simulink model "receiver"  (R2020b)
settings: Solver=VariableStepAuto  StartTime=0.0  StopTime=10000/3.2e6  RelTol=1e-3
PreLoadFcn:
  | setup_receiver
InitFcn:
  | setup_receiver
undefined symbols (not defined in the file): AXI4, designMultirateFIR, fir_bbuf, Lite, tx_data, xlfda_numerator
libraries: xbsIndex_r4 x428, hdlsllib x13, dspmlti4 x8, xrbsSSR_Library x6, dspswit3 x4, commrandsrc3 x2, dspsigops x2, simulink x1
(part 3 of 5)

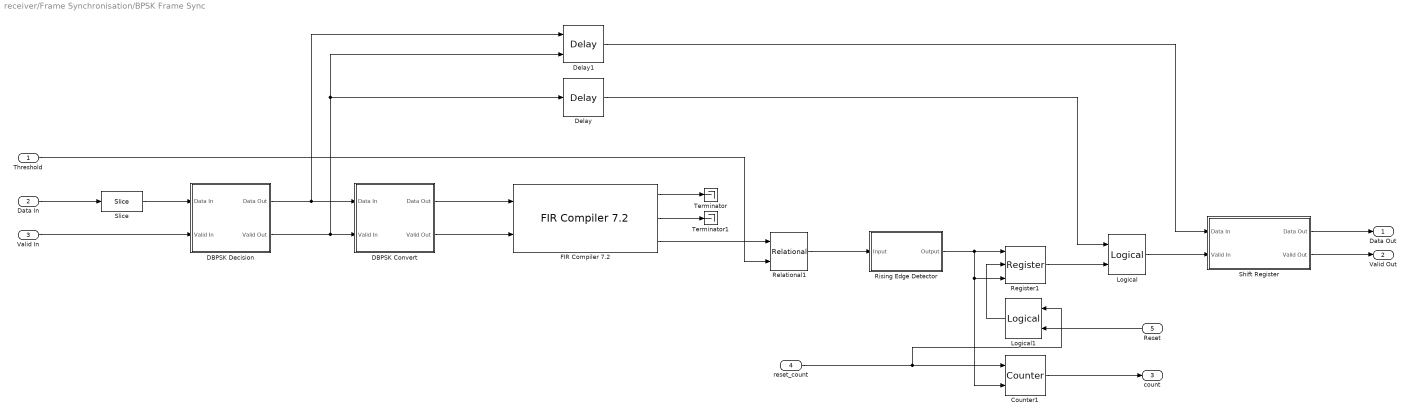
== system receiver/Frame Synchronisation/BPSK Frame Sync ==
  Threshold : Inport
  Data In : Inport  Port=2
  Valid In : Inport  Port=3
  reset_count : Inport  Port=4
  Reset : Inport  Port=5
  Counter1 : xbsIndex_r4/Counter  cnt_type=Free Running  cnt_to=Inf  operation=Up  start_count=0  cnt_by_val=1  arith_type=Unsigned  n_bits=32  bin_pt=0  load_pin=off  rst=on  en=on  explicit_period=off  period=1  use_behavioral_HDL=off  implementation=Fabric  dbl_ovrd=off  block_type=counter
  DBPSK Convert : Subsystem
  DBPSK Decision : Subsystem
  Delay : xbsIndex_r4/Delay  rst=off  infoeditControl=Selection of Reset will increase slice count due to use of real FFs and instead of SRLs  en=off  latency=2  reg_retiming=off  dbl_ovrd=off  block_type=delay
  Delay1 : xbsIndex_r4/Delay  rst=off  infoeditControl=Selection of Reset will increase slice count due to use of real FFs and instead of SRLs  en=on  latency=2  reg_retiming=off  dbl_ovrd=off  block_type=delay
  "FIR Compiler 7.2 " : xbsIndex_r4/FIR Compiler 7.2   coefficientvector=fliplr(double(fir_bbuf))  coefficient_sets=1  coefficient_reload=off  filter_type=Single_Rate  rate_change_type=Integer  interpolation_rate=1  decimation_rate=1  zero_pack_factor=1  channel_sequence=Basic  number_channels=1  pattern_list='P4-0,P4-1,P4-2,P4-3,P4-4'  number_paths=1  ratespecification=Maximum_Possible  sampleperiod=40  hardwareoversamplingrate=1  coefficient_sign=Signed  quantization=Integer_Coefficients  coefficient_width=2  bestprecision=off  coefficient_fractional_bits=0  coefficient_structure=Inferred  output_rounding_mode=Full_Precision  output_width=22  filter_architecture=Systolic_Multiply_Accumulate  optimization_goal=Area  optimization_list='None'  data_buffer_type=Automatic  coefficient_buffer_type=Automatic  input_buffer_type=Automatic  output_buffer_type=Automatic  preference_for_other_storage=Automatic  multi_column_support=Automatic  columnconfig='39'  inter_column_pipe_length=4  data_has_tlast=Not_Required  m_data_has_tready=off  s_data_has_fifo=off  s_data_has_tuser=Not_Required  m_data_has_tuser=Not_Required  s_config_sync_mode=On_Vector  s_config_method=Single  num_reload_slots=1  has_aclken=on  has_aresetn=off  infoeditControl=ARESETn must be asserted for a minimum of 2 cycles  reset_data_vector=on  trim_axipin_name=on  simulation_type=hybrid_sim  simulation_model=sysgen:xfirv7_2_cmodel  data_path_portlist={ 's_axis_data_tdata', 'm_axis_data_tdata' }  passband_min=0.0  passband_max=0.5  stopband_min=0.5  stopband_max=1.0  filter_selection=1  gui_behaviour='Sysgen_GUI'  data_sign=Signed  data_width=16  data_fractional_bits=0  data_tuser_width=1  wrapper_available=true  ip_wrap_arbitrary_binary_point=true  ip_name=FIR Compiler  ip_version=7.2  dsptool_ready=true  ipcore_usecache=true  ipcore_useipmodelcache=true  port_translation_map={ 'aclken' => 'en', 'aresetn' => 'rst' }  run_core_at_system_period=true  ipcore_xco_need_fpga_part=true  block_type=fir_compiler_v7_2
      settings: infoedit=Maximum Possible : Maximizes oversampling rate. Abstracted input handshake (no s_data_tvalid) and automatic rate propagation.<br>Hardware Oversampling Rate : Specifies oversampling rate relative to the input sample period. Abstracted input handshake (no s_data_tvalid) and automatic rate propagation.<br>Input/Output Sample Period : Specifies absolute oversampling rate. No input handshake abstraction (exposes s_data_tvalid) and no rate propagation.
  Logical : xbsIndex_r4/Logical  logical_function=AND  inputs=2  en=off  latency=0  precision=Full  arith_type=Unsigned  n_bits=16  bin_pt=0  align_bp=on  dbl_ovrd=off  block_type=logical
  Logical1 : xbsIndex_r4/Logical  logical_function=OR  inputs=2  en=off  latency=0  precision=Full  arith_type=Unsigned  n_bits=16  bin_pt=0  align_bp=on  dbl_ovrd=off  block_type=logical
  Register1 : xbsIndex_r4/Register  init=0  rst=on  en=on  dbl_ovrd=off  block_type=register
  Relational1 : xbsIndex_r4/Relational  mode=a>=b  op_type=Bool  en=off  latency=0  dbl_ovrd=off  block_type=relational
  Rising Edge Detector : Subsystem
  Shift Register : Subsystem
  Slice : xbsIndex_r4/Slice  nbits=1  boolean_output=off  mode=Upper Bit Location + Width  bit1=0  base1=MSB of Input  bit0=0  base0=LSB of Input  dbl_ovrd=off  block_type=slice
  Terminator : Terminator
  Terminator1 : Terminator
  Data Out : Outport  VectorParamsAs1DForOutWhenUnconnected=off
  Valid Out : Outport  Port=2  VectorParamsAs1DForOutWhenUnconnected=off
  count : Outport  Port=3  VectorParamsAs1DForOutWhenUnconnected=off
  wires:
  DBPSK Convert/1(Data Out) -> "FIR Compiler 7.2 "/1
  DBPSK Decision/2(Valid Out) -> Delay1/2, Delay/1, DBPSK Convert/2(Valid In)
  Reset/1 -> Logical1/2
  Relational1/1 -> Rising Edge Detector/1(Input)
  DBPSK Decision/1(Data Out) -> Delay1/1, DBPSK Convert/1(Data In)
  Delay1/1 -> Shift Register/1(Data In)
  Logical/1 -> Shift Register/2(Valid In)
  Threshold/1 -> Relational1/2
  Logical1/1 -> Register1/2
  Counter1/1 -> count/1
  Valid In/1 -> DBPSK Decision/2(Valid In)
  Slice/1 -> DBPSK Decision/1(Data In)
  "FIR Compiler 7.2 "/2 -> Terminator1/1
  Rising Edge Detector/1(Output) -> Counter1/2, Register1/3, Register1/1
  Register1/1 -> Logical/2
  Shift Register/1(Data Out) -> Data Out/1
  DBPSK Convert/2(Valid Out) -> "FIR Compiler 7.2 "/2
  "FIR Compiler 7.2 "/1 -> Terminator/1
  reset_count/1 -> Logical1/1, Counter1/1
  "FIR Compiler 7.2 "/3 -> Relational1/1
  Delay/1 -> Logical/1
  Data In/1 -> Slice/1
  Shift Register/2(Valid Out) -> Valid Out/1

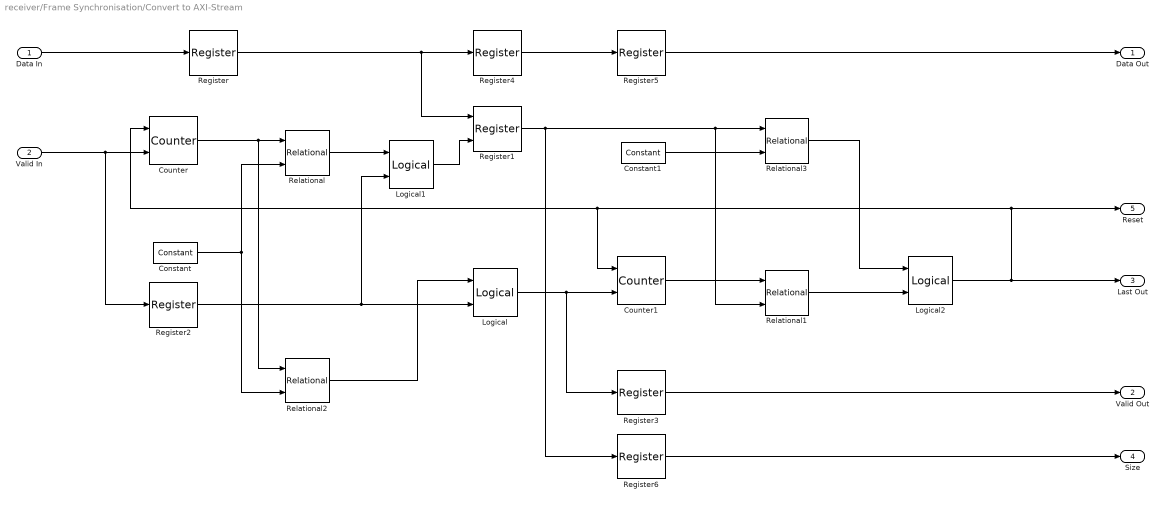
== system receiver/Frame Synchronisation/Convert to AXI-Stream ==
  Data In : Inport
  Valid In : Inport  Port=2
  Constant : xbsIndex_r4/Constant  const=1.0  gui_display_data_type=Fixed-point  arith_type=Unsigned  n_bits=1  bin_pt=0  preci_type=Single  exp_width=8  frac_width=24  explicit_period=off  period=1  equ=P=C  opselect=C  inp2=PCIN>>17  opr=+  inp1=P  carry=CIN  dbl_ovrd=off  block_type=constant
  Constant1 : xbsIndex_r4/Constant  const=0  gui_display_data_type=Fixed-point  arith_type=Unsigned  n_bits=1  bin_pt=0  preci_type=Single  exp_width=8  frac_width=24  explicit_period=off  period=1  equ=P=C  opselect=C  inp2=PCIN>>17  opr=+  inp1=P  carry=CIN  dbl_ovrd=off  block_type=constant
  Counter : xbsIndex_r4/Counter  cnt_type=Free Running  cnt_to=Inf  operation=Up  start_count=0  cnt_by_val=1  arith_type=Unsigned  n_bits=32  bin_pt=0  load_pin=off  rst=on  en=on  explicit_period=off  period=1  use_behavioral_HDL=off  implementation=Fabric  dbl_ovrd=off  block_type=counter
  Counter1 : xbsIndex_r4/Counter  cnt_type=Free Running  cnt_to=Inf  operation=Up  start_count=0  cnt_by_val=1  arith_type=Unsigned  n_bits=32  bin_pt=0  load_pin=off  rst=on  en=on  explicit_period=off  period=1  use_behavioral_HDL=off  implementation=Fabric  dbl_ovrd=off  block_type=counter
  Logical : xbsIndex_r4/Logical  logical_function=AND  inputs=2  en=off  latency=1  precision=Full  arith_type=Unsigned  n_bits=16  bin_pt=0  align_bp=on  dbl_ovrd=off  block_type=logical
  Logical1 : xbsIndex_r4/Logical  logical_function=AND  inputs=2  en=off  latency=0  precision=Full  arith_type=Unsigned  n_bits=16  bin_pt=0  align_bp=on  dbl_ovrd=off  block_type=logical
  Logical2 : xbsIndex_r4/Logical  logical_function=AND  inputs=2  en=off  latency=0  precision=Full  arith_type=Unsigned  n_bits=16  bin_pt=0  align_bp=on  dbl_ovrd=off  block_type=logical
  Register{,2..6} (6 alike) : xbsIndex_r4/Register  init=0  rst=off  en=off  dbl_ovrd=off  block_type=register
  Register1 : xbsIndex_r4/Register  init=0  rst=off  en=on  dbl_ovrd=off  block_type=register
  Relational : xbsIndex_r4/Relational  mode=a=b  op_type=Bool  en=off  latency=0  dbl_ovrd=off  block_type=relational
  Relational1 : xbsIndex_r4/Relational  mode=a>=b  op_type=Bool  en=off  latency=0  dbl_ovrd=off  block_type=relational
  Relational2 : xbsIndex_r4/Relational  mode=a>b  op_type=Bool  en=off  latency=0  dbl_ovrd=off  block_type=relational
  Relational3 : xbsIndex_r4/Relational  mode=a!=b  op_type=Bool  en=off  latency=0  dbl_ovrd=off  block_type=relational
  Data Out : Outport  VectorParamsAs1DForOutWhenUnconnected=off
  Valid Out : Outport  Port=2  VectorParamsAs1DForOutWhenUnconnected=off
  Last Out : Outport  Port=3  VectorParamsAs1DForOutWhenUnconnected=off
  Size : Outport  Port=4  VectorParamsAs1DForOutWhenUnconnected=off
  Reset : Outport  Port=5  VectorParamsAs1DForOutWhenUnconnected=off
  wires:
  Valid In/1 -> Register2/1, Counter/2
  Counter/1 -> Relational2/1, Relational/1
  Data In/1 -> Register/1
  Register/1 -> Register4/1, Register1/1
  Logical/1 -> Register3/1, Counter1/2
  Counter1/1 -> Relational1/1
  Register1/1 -> Register6/1, Relational3/1, Relational1/2
  Register2/1 -> Logical1/2, Logical/2
  Register3/1 -> Valid Out/1
  Register4/1 -> Register5/1
  Register5/1 -> Data Out/1
  Constant/1 -> Relational/2, Relational2/2
  Relational2/1 -> Logical/1
  Relational/1 -> Logical1/1
  Logical1/1 -> Register1/2
  Constant1/1 -> Relational3/2
  Relational3/1 -> Logical2/1
  Relational1/1 -> Logical2/2
  Logical2/1 -> Counter/1, Counter1/1, Reset/1, Last Out/1
  Register6/1 -> Size/1

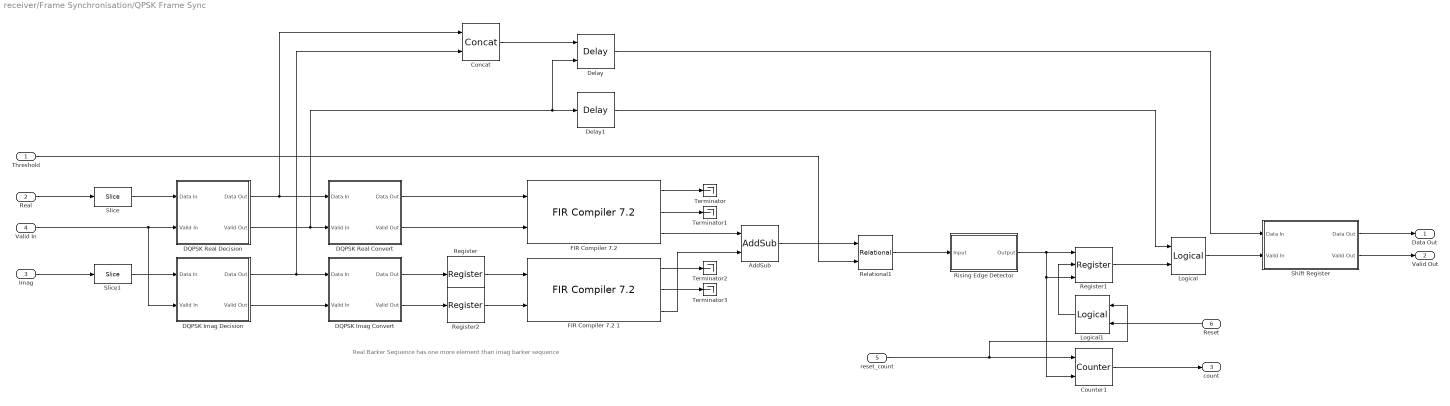
== system receiver/Frame Synchronisation/QPSK Frame Sync ==
  note: Real Barker Sequence has one more element than imag barker sequence
  Threshold : Inport
  Real : Inport  Port=2
  Imag : Inport  Port=3
  Valid In : Inport  Port=4
  reset_count : Inport  Port=5
  Reset : Inport  Port=6
  AddSub : xbsIndex_r4/AddSub  mode=Addition  use_carryin=off  use_carryout=off  en=off  latency=0  precision=Full  arith_type=Unsigned  n_bits=16  bin_pt=14  quantization=Truncate  overflow=Wrap  use_behavioral_HDL=off  hw_selection=Fabric  pipelined=off  dbl_ovrd=off  block_type=addsub
  Concat : xbsIndex_r4/Concat  num_inputs=2  dbl_ovrd=off  block_type=concat
  Counter1 : xbsIndex_r4/Counter  cnt_type=Free Running  cnt_to=Inf  operation=Up  start_count=0  cnt_by_val=1  arith_type=Unsigned  n_bits=32  bin_pt=0  load_pin=off  rst=on  en=on  explicit_period=off  period=1  use_behavioral_HDL=off  implementation=Fabric  dbl_ovrd=off  block_type=counter
  DQPSK Imag Convert : Subsystem
  DQPSK Imag Decision : Subsystem
  DQPSK Real Convert : Subsystem
  DQPSK Real Decision : Subsystem
  Delay : xbsIndex_r4/Delay  rst=off  infoeditControl=Selection of Reset will increase slice count due to use of real FFs and instead of SRLs  en=on  latency=3  reg_retiming=off  dbl_ovrd=off  block_type=delay
  Delay1 : xbsIndex_r4/Delay  rst=off  infoeditControl=Selection of Reset will increase slice count due to use of real FFs and instead of SRLs  en=off  latency=1  reg_retiming=off  dbl_ovrd=off  block_type=delay
  "FIR Compiler 7.2 " : xbsIndex_r4/FIR Compiler 7.2   coefficientvector=fliplr(double(fir_bbuf(1:2:end)))  coefficient_sets=1  coefficient_reload=off  filter_type=Single_Rate  rate_change_type=Integer  interpolation_rate=1  decimation_rate=1  zero_pack_factor=1  channel_sequence=Basic  number_channels=1  pattern_list='P4-0,P4-1,P4-2,P4-3,P4-4'  number_paths=1  ratespecification=Maximum_Possible  sampleperiod=20  hardwareoversamplingrate=1  coefficient_sign=Signed  quantization=Integer_Coefficients  coefficient_width=2  bestprecision=off  coefficient_fractional_bits=0  coefficient_structure=Inferred  output_rounding_mode=Full_Precision  output_width=21  filter_architecture=Systolic_Multiply_Accumulate  optimization_goal=Area  optimization_list='None'  data_buffer_type=Automatic  coefficient_buffer_type=Automatic  input_buffer_type=Automatic  output_buffer_type=Automatic  preference_for_other_storage=Automatic  multi_column_support=Automatic  columnconfig='20'  inter_column_pipe_length=4  data_has_tlast=Not_Required  m_data_has_tready=off  s_data_has_fifo=off  s_data_has_tuser=Not_Required  m_data_has_tuser=Not_Required  s_config_sync_mode=On_Vector  s_config_method=Single  num_reload_slots=1  has_aclken=on  has_aresetn=off  infoeditControl=ARESETn must be asserted for a minimum of 2 cycles  reset_data_vector=on  trim_axipin_name=on  simulation_type=hybrid_sim  simulation_model=sysgen:xfirv7_2_cmodel  data_path_portlist={ 's_axis_data_tdata', 'm_axis_data_tdata' }  passband_min=0.0  passband_max=0.5  stopband_min=0.5  stopband_max=1.0  filter_selection=1  gui_behaviour='Sysgen_GUI'  data_sign=Signed  data_width=16  data_fractional_bits=0  data_tuser_width=1  wrapper_available=true  ip_wrap_arbitrary_binary_point=true  ip_name=FIR Compiler  ip_version=7.2  dsptool_ready=true  ipcore_usecache=true  ipcore_useipmodelcache=true  port_translation_map={ 'aclken' => 'en', 'aresetn' => 'rst' }  run_core_at_system_period=true  ipcore_xco_need_fpga_part=true  block_type=fir_compiler_v7_2
      settings: infoedit=Maximum Possible : Maximizes oversampling rate. Abstracted input handshake (no s_data_tvalid) and automatic rate propagation.<br>Hardware Oversampling Rate : Specifies oversampling rate relative to the input sample period. Abstracted input handshake (no s_data_tvalid) and automatic rate propagation.<br>Input/Output Sample Period : Specifies absolute oversampling rate. No input handshake abstraction (exposes s_data_tvalid) and no rate propagation.
  FIR Compiler 7.2 1 : xbsIndex_r4/FIR Compiler 7.2   coefficientvector=fliplr(double(fir_bbuf(2:2:end)))  coefficient_sets=1  coefficient_reload=off  filter_type=Single_Rate  rate_change_type=Integer  interpolation_rate=1  decimation_rate=1  zero_pack_factor=1  channel_sequence=Basic  number_channels=1  pattern_list='P4-0,P4-1,P4-2,P4-3,P4-4'  number_paths=1  ratespecification=Maximum_Possible  sampleperiod=20  hardwareoversamplingrate=1  coefficient_sign=Signed  quantization=Integer_Coefficients  coefficient_width=2  bestprecision=off  coefficient_fractional_bits=0  coefficient_structure=Inferred  output_rounding_mode=Full_Precision  output_width=21  filter_architecture=Systolic_Multiply_Accumulate  optimization_goal=Area  optimization_list='None'  data_buffer_type=Automatic  coefficient_buffer_type=Automatic  input_buffer_type=Automatic  output_buffer_type=Automatic  preference_for_other_storage=Automatic  multi_column_support=Automatic  columnconfig='19'  inter_column_pipe_length=4  data_has_tlast=Not_Required  m_data_has_tready=off  s_data_has_fifo=off  s_data_has_tuser=Not_Required  m_data_has_tuser=Not_Required  s_config_sync_mode=On_Vector  s_config_method=Single  num_reload_slots=1  has_aclken=on  has_aresetn=off  infoeditControl=ARESETn must be asserted for a minimum of 2 cycles  reset_data_vector=on  trim_axipin_name=on  simulation_type=hybrid_sim  simulation_model=sysgen:xfirv7_2_cmodel  data_path_portlist={ 's_axis_data_tdata', 'm_axis_data_tdata' }  passband_min=0.0  passband_max=0.5  stopband_min=0.5  stopband_max=1.0  filter_selection=1  gui_behaviour='Sysgen_GUI'  data_sign=Signed  data_width=16  data_fractional_bits=0  data_tuser_width=1  wrapper_available=true  ip_wrap_arbitrary_binary_point=true  ip_name=FIR Compiler  ip_version=7.2  dsptool_ready=true  ipcore_usecache=true  ipcore_useipmodelcache=true  port_translation_map={ 'aclken' => 'en', 'aresetn' => 'rst' }  run_core_at_system_period=true  ipcore_xco_need_fpga_part=true  block_type=fir_compiler_v7_2
      settings: infoedit=Maximum Possible : Maximizes oversampling rate. Abstracted input handshake (no s_data_tvalid) and automatic rate propagation.<br>Hardware Oversampling Rate : Specifies oversampling rate relative to the input sample period. Abstracted input handshake (no s_data_tvalid) and automatic rate propagation.<br>Input/Output Sample Period : Specifies absolute oversampling rate. No input handshake abstraction (exposes s_data_tvalid) and no rate propagation.
  Logical : xbsIndex_r4/Logical  logical_function=AND  inputs=2  en=off  latency=0  precision=Full  arith_type=Unsigned  n_bits=16  bin_pt=0  align_bp=on  dbl_ovrd=off  block_type=logical
  Logical1 : xbsIndex_r4/Logical  logical_function=OR  inputs=2  en=off  latency=0  precision=Full  arith_type=Unsigned  n_bits=16  bin_pt=0  align_bp=on  dbl_ovrd=off  block_type=logical
  Register : xbsIndex_r4/Register  init=0  rst=off  en=off  dbl_ovrd=off  block_type=register
  Register1 : xbsIndex_r4/Register  init=0  rst=on  en=on  dbl_ovrd=off  block_type=register
  Register2 : xbsIndex_r4/Register  init=0  rst=off  en=off  dbl_ovrd=off  block_type=register
  Relational1 : xbsIndex_r4/Relational  mode=a>=b  op_type=Bool  en=off  latency=0  dbl_ovrd=off  block_type=relational
  Rising Edge Detector : Subsystem
  Shift Register : Subsystem
  Slice : xbsIndex_r4/Slice  nbits=1  boolean_output=off  mode=Upper Bit Location + Width  bit1=0  base1=MSB of Input  bit0=0  base0=LSB of Input  dbl_ovrd=off  block_type=slice
  Slice1 : xbsIndex_r4/Slice  nbits=1  boolean_output=off  mode=Upper Bit Location + Width  bit1=0  base1=MSB of Input  bit0=0  base0=LSB of Input  dbl_ovrd=off  block_type=slice
  Terminator{,1..3} (4 alike) : Terminator
  Data Out : Outport  VectorParamsAs1DForOutWhenUnconnected=off
  Valid Out : Outport  Port=2  VectorParamsAs1DForOutWhenUnconnected=off
  count : Outport  Port=3  VectorParamsAs1DForOutWhenUnconnected=off
  wires:
  Delay1/1 -> Logical/1
  Delay/1 -> Shift Register/1(Data In)
  Concat/1 -> Delay/1
  Register2/1 -> FIR Compiler 7.2 1/2
  Register/1 -> FIR Compiler 7.2 1/1
  DQPSK Imag Convert/2(Valid Out) -> Register2/1
  DQPSK Imag Convert/1(Data Out) -> Register/1
  FIR Compiler 7.2 1/1 -> Terminator2/1
  FIR Compiler 7.2 1/2 -> Terminator3/1
  FIR Compiler 7.2 1/3 -> AddSub/2
  AddSub/1 -> Relational1/1
  "FIR Compiler 7.2 "/3 -> AddSub/1
  DQPSK Imag Decision/2(Valid Out) -> DQPSK Imag Convert/2(Valid In)
  DQPSK Imag Decision/1(Data Out) -> DQPSK Imag Convert/1(Data In), Concat/2
  Slice1/1 -> DQPSK Imag Decision/1(Data In)
  Imag/1 -> Slice1/1
  DQPSK Real Convert/1(Data Out) -> "FIR Compiler 7.2 "/1
  Reset/1 -> Logical1/2
  Relational1/1 -> Rising Edge Detector/1(Input)
  DQPSK Real Decision/1(Data Out) -> DQPSK Real Convert/1(Data In), Concat/1
  Logical/1 -> Shift Register/2(Valid In)
  Threshold/1 -> Relational1/2
  Logical1/1 -> Register1/2
  Counter1/1 -> count/1
  Valid In/1 -> DQPSK Real Decision/2(Valid In), DQPSK Imag Decision/2(Valid In)
  Slice/1 -> DQPSK Real Decision/1(Data In)
  "FIR Compiler 7.2 "/2 -> Terminator1/1
  Rising Edge Detector/1(Output) -> Counter1/2, Register1/3, Register1/1
  Register1/1 -> Logical/2
  Shift Register/1(Data Out) -> Data Out/1
  DQPSK Real Convert/2(Valid Out) -> "FIR Compiler 7.2 "/2
  "FIR Compiler 7.2 "/1 -> Terminator/1
  reset_count/1 -> Logical1/1, Counter1/1
  DQPSK Real Decision/2(Valid Out) -> DQPSK Real Convert/2(Valid In), Delay1/1, Delay/2
  Real/1 -> Slice/1
  Shift Register/2(Valid Out) -> Valid Out/1

== system receiver/Observation Point/op ==
  Data In : Inport
  Valid In : Inport  Port=2
  Cast To Boolean : DataTypeConversion  OutDataTypeStr=boolean
  Constellation Diagram : ConstellationDiagram
  Convert Protect : DataTypeConversion  OutDataTypeStr=fixdt(0,32,0)  ConvertRealWorld=Stored Integer (SI)
  Delay : Delay  DelayLength=1  ShowEnablePort=on
      settings: InputPortMap=u0,e6
  Imag Conversion : DataTypeConversion  OutDataTypeStr=fixdt(1,16,15)  ConvertRealWorld=Stored Integer (SI)
  Imag Slice : hdlsllib/Logic and Bit Operations/Bit Slice  lidx=31  ridx=16
      settings: SourceProductBaseCode=SL
  Real Conversion : DataTypeConversion  OutDataTypeStr=fixdt(1,16,15)  ConvertRealWorld=Stored Integer (SI)
  Real Slice : hdlsllib/Logic and Bit Operations/Bit Slice  lidx=15  ridx=0
      settings: SourceProductBaseCode=SL
  Real-Imag to Complex : RealImagToComplex
  Time Scope : Scope
  m_axis_op_tdata : xbsIndex_r4/Gateway Out  inherit_from_input=on  hdl_port=on  rows=1  columns=1  UseAsDAC=off  DACChannel='1'  interface=None  automatic_assignment=on  address_offset=hex2dec('00')  intf_name=''  intf_description=''  timing_constraint=None  locs_specified=off  LOCs={}  io_standard={}  block_type=gatewayout
  m_axis_op_tvalid : xbsIndex_r4/Gateway Out  inherit_from_input=on  hdl_port=on  rows=1  columns=1  UseAsDAC=off  DACChannel='1'  interface=None  automatic_assignment=on  address_offset=hex2dec('00')  intf_name=''  intf_description=''  timing_constraint=None  locs_specified=off  LOCs={}  io_standard={}  block_type=gatewayout
  wires:
  Cast To Boolean/1 -> Delay/2
  Convert Protect/1 -> Imag Slice/1, Real Slice/1
  Real-Imag to Complex/1 -> Delay/1
  m_axis_op_tdata/1 -> Convert Protect/1
  Imag Conversion/1 -> Real-Imag to Complex/2
  Imag Slice/1 -> Imag Conversion/1
  Real Slice/1 -> Real Conversion/1
  Real Conversion/1 -> Real-Imag to Complex/1
  m_axis_op_tvalid/1 -> Cast To Boolean/1
  Delay/1 -> Constellation Diagram/1, Time Scope/1
  Data In/1 -> m_axis_op_tdata/1
  Valid In/1 -> m_axis_op_tvalid/1

== system receiver/QPSK System/QPSK TX Generation ==
  Enable : Inport
  Bernoulli Binary Generator : commrandsrc3/Bernoulli Binary Generator  ProbabilityOfZero=0.5  SeedSource=Parameter  Seed=53  SampleTime=1/100e3  SamplesPerFrame=1  OutputDataType=double  SimulateUsing=Interpreted execution
  Bernoulli Binary Generator1 : commrandsrc3/Bernoulli Binary Generator  ProbabilityOfZero=0.5  SeedSource=Parameter  Seed=1  SampleTime=1/100e3  SamplesPerFrame=1  OutputDataType=double  SimulateUsing=Interpreted execution
  CIC Interpolation : dspmlti4/CIC Interpolation  filtFrom=Dialog parameters  filtobj=Hm_interp  ftype=Interpolator  R=320  M=1  N=5  filterInternals=Full precision  BPS=[16 16 16 16]  FLPS=0  outputWordLength=32  outputFracLength=0  launchFVT=off  framing=Allow multirate processing  OutputFrames=off
      settings: SourceProductBaseCode=DS
  Constant : Constant  SampleTime=1/25e3
  DMA Read : Subsystem
  DQPSK Modulator : Subsystem
  Data Type Conversion2 : DataTypeConversion  OutDataTypeStr=fixdt(1,16,14)
  FDATool : xbsIndex_r4/FDATool  block_type=fdatool
      settings: infoedit=FDATool
  FIR Interpolation : dspmlti4/FIR Interpolation  FilterSource=Dialog parameters  PrivateCoeffs=0  h=xlfda_numerator('FDATool')*4  L=4  FilterObject=xlfda_numerator('FDATool')/(max(xlfda_numerator('FDATool')))  framing=Allow multirate processing  outputBufInitCond=0  roundingMode=Floor  overflowMode=off  firstCoeffMode=Binary point scaling  firstCoeffWordLength=16  firstCoeffFracLength=14  firstCoeffDataTypeStr=fixdt(1,16,14)  firstCoeffMin=[]  firstCoeffMax=[]  firstCoeffLastDataTypeStr=fixdt(1,16,14)  outputDataTypeStr=Inherit: Same as accumulator  outputMin=[]  outputMax=[]  outputLastDataTypeStr=Inherit: Same as accumulator
  Multiply : Gain  Gain=fi(0.8192, 1, 16, 14)  ParamDataTypeStr=fixdt(1,16,15)  OutDataTypeStr=fixdt(1,16,14)
  Multiply1 : Gain  Gain=0.75  ParamDataTypeStr=double  OutDataTypeStr=fixdt(1,16,14)
  Multiport Switch : MultiPortSwitch  DataPortOrder=Zero-based contiguous  Inputs=2  zeroidx=on
  Real-Imag to Complex : RealImagToComplex
  Shift Arithmetic : ArithShift  BitShiftNumber=33  BitShiftDirection=Right
  Terminator1 : Terminator
  QPSK : Outport  VectorParamsAs1DForOutWhenUnconnected=off
  wires:
  Multiply1/1 -> QPSK/1
  Multiply/1 -> Multiply1/1
  Shift Arithmetic/1 -> Multiply/1
  Data Type Conversion2/1 -> CIC Interpolation/1
  DQPSK Modulator/1(Output) -> FIR Interpolation/1
  Multiport Switch/1 -> DQPSK Modulator/1(Input)
  Constant/1 -> DMA Read/2(tready)
  Enable/1 -> DMA Read/1(enable)
  DMA Read/3(tlast) -> Terminator1/1
  DMA Read/1(tdata) -> Multiport Switch/3
  DMA Read/2(tvalid) -> Multiport Switch/1
  FIR Interpolation/1 -> Data Type Conversion2/1
  CIC Interpolation/1 -> Shift Arithmetic/1
  Bernoulli Binary Generator1/1 -> Real-Imag to Complex/1
  Bernoulli Binary Generator/1 -> Real-Imag to Complex/2
  Real-Imag to Complex/1 -> Multiport Switch/2

== system receiver/QPSK System/RF-ADC ==
  Data In : Inport
  Decimation Filter : Subsystem  mask{decim=8x}
      mask prompts: decim "Decimation Factor:"
      mask init:
      | fir0 = dsp.FIRDecimator('DecimationFactor', 2,...
      |                            'CoefficientsDataType', 'Custom',...
      |                            'CustomCoefficientsDataType', numerictype([], 16, 14),...
      |                            'FullPrecisionOverride', false,...
      |                            'OutputDataType', 'Custom',...
      |                            'CustomOutputDataType', numerictype([], 16, 14),...
      |                            'Numerator', [-6, 0 54, 0, -254, 0, 1230, 2048, 1230, 0, -254, 0, 54, 0, -6]/(2048*2));
      | fir1 = dsp.FIRDecimator('DecimationFactor', 2,...
      |                            'CoefficientsDataType', 'Custom',...
      |                            'CustomCoefficientsDataType', numerictype([], 16, 14),...
      |                            'FullPrecisionOverride', false,...
      |                            'OutputDataType', 'Custom',...
      |                            'CustomOutputDataType', numerictype([], 16, 14),...
      |                            'Numerator', [-12, 0, 84, 0, -337, 0, 1008, 0, -2693, 0, 10142, 16384, 10142, 0, -2693, 0, 1008, 0, -337, 0, 84, 0 ,-12]/(16384*2));
      | fir2 = dsp.FIRDecimator('DecimationFactor', 2,...
      |                            'CoefficientsDataType', 'Custom',...
      |                            'CustomCoefficientsDataType', numerictype([], 16, 14),...
      |                            'FullPrecisionOverride', false,...
      |                            'OutputDataType', 'Custom',...
      |                            'CustomOutputDataType', numerictype([], 16, 14),...
      |                            'Numerator', [5, 0, -17, 0, 44, 0, -96, 0, 187, 0, -335, 0, 565, 0, -906, 0, 1401, 0, -2112, 0, 3145, 0, -4723, 0, 7415, 0, -13331, 0, 41526, 65536, 41526, 0, -13331, 0, 7415, 0, -4723, 0, 3145, 0, -2112, 0, 1401, 0, -906, 0, 565, 0, -335, 0, 187, 0, -96, 0, 44, 0, -17, 0, 5]/(65536));
      | switch get_param(gcb, 'decim')
      |     case '1x'
      |         if ~strcmp(get_param([gcb, '/FIR 0'], 'Commented'), 'through')
      |             set_param([gcb, '/FIR 0'],'Commented','through');
      |         end
      |         
      |         if ~strcmp(get_param([gcb, '/FIR 1'], 'Commented'), 'through')
      |             set_param([gcb, '/FIR 1'],'Commented','through');
      |         end
      |         
      |         if ~strcmp(get_param([gcb, '/FIR 2'], 'Commented'), 'through')
      |             set_param([gcb, '/FIR 2'],'Commented','through');
      |         end
      |             
      |     case '2x'
      |         if ~strcmp(get_param([gcb, '/FIR 0'], 'Commented'), 'through')
      |             set_param([gcb, '/FIR 0'],'Commented','through');
      |         end
      |         
      |         if ~strcmp(get_param([gcb, '/FIR 1'], 'Commented'), 'through')
      |             set_param([gcb, '/FIR 1'],'Commented','through');
      |         end
      |         
      |         if ~strcmp(get_param([gcb, '/FIR 2'], 'Commented'), 'off')
      |             set_param([gcb, '/FIR 2'],'Commented','off');
      |         end
      | 
      |     case '4x'
      |         if ~strcmp(get_param([gcb, '/FIR 0'], 'Commented'), 'through')
      |             set_param([gcb, '/FIR 0'],'Commented','through');
      |         end
      |         
      |         if ~strcmp(get_param([gcb, '/FIR 1'], 'Commented'), 'off')
      |             set_param([gcb, '/FIR 1'],'Commented','off');
      |         end
      |         
      |         if ~strcmp(get_param([gcb, '/FIR 2'], 'Commented'), 'off')
      |             set_param([gcb, '/FIR 2'],'Commented','off');
      |         end
      |         
      |     case '8x'
      |         if ~strcmp(get_param([gcb, '/FIR 0'], 'Commented'), 'off')
      |             set_param([gcb, '/FIR 0'],'Commented','off');
      |         end
      |         
      |         if ~strcmp(get_param([gcb, '/FIR 1'], 'Commented'), 'off')
      |             set_param([gcb, '/FIR 1'],'Commented','off');
      |         end
      |         
      |         if ~strcmp(get_param([gcb, '/FIR 2'], 'Commented'), 'off')
      |             set_param([gcb, '/FIR 2'],'Commented','off');
      |         end
      | 
      | end
      mask TypeOptions decim: 1x | 2x | 4x | 8x
      mask DialogControl DescGroupVar Prompt: RF-DAC Interpolation Filter
      mask DialogControl DescTextVar Prompt: This block simulates the RF-DAC interpolation stage using the same coefficients stored in the interpolation filters.
      mask DialogControl ParameterGroupVar Prompt: Main
  NCO and Mixer : Subsystem
  RF-ADC : Subsystem
  Data Out : Outport  VectorParamsAs1DForOutWhenUnconnected=off
  wires:
  NCO and Mixer/1(Data Out) -> Decimation Filter/1(Data In)
  RF-ADC/1(Data Out) -> NCO and Mixer/1(Data In)
  Data In/1 -> RF-ADC/1(Data In)
  Decimation Filter/1(Data Out) -> Data Out/1

== system receiver/QPSK System/RF-DAC ==
  note: Not Ready
  Data In : Inport
  Coarse Delay : Subsystem
  Interpolation Filter : Subsystem  mask{interp=8x}
      mask prompts: interp "Interpolation Factor:"
      mask init:
      | fir0 = dsp.FIRInterpolator('InterpolationFactor', 2,...
      |                            'CoefficientsDataType', 'Custom',...
      |                            'CustomCoefficientsDataType', numerictype([], 16, 14),...
      |                            'FullPrecisionOverride', false,...
      |                            'OutputDataType', 'Custom',...
      |                            'CustomOutputDataType', numerictype([], 16, 14),...
      |                            'Numerator', [-6, 0 54, 0, -254, 0, 1230, 2048, 1230, 0, -254, 0, 54, 0, -6]/(2048));
      | fir1 = dsp.FIRInterpolator('InterpolationFactor', 2,...
      |                            'CoefficientsDataType', 'Custom',...
      |                            'CustomCoefficientsDataType', numerictype([], 16, 14),...
      |                            'FullPrecisionOverride', false,...
      |                            'OutputDataType', 'Custom',...
      |                            'CustomOutputDataType', numerictype([], 16, 14),...
      |                            'Numerator', [-12, 0, 84, 0, -337, 0, 1008, 0, -2693, 0, 10142, 16384, 10142, 0, -2693, 0, 1008, 0, -337, 0, 84, 0 ,-12]/(16384));
      | fir2 = dsp.FIRInterpolator('InterpolationFactor', 2,...
      |                            'CoefficientsDataType', 'Custom',...
      |                            'CustomCoefficientsDataType', numerictype([], 16, 14),...
      |                            'FullPrecisionOverride', false,...
      |                            'OutputDataType', 'Custom',...
      |                            'CustomOutputDataType', numerictype([], 16, 14),...
      |                            'Numerator', [5, 0, -17, 0, 44, 0, -96, 0, 187, 0, -335, 0, 565, 0, -906, 0, 1401, 0, -2112, 0, 3145, 0, -4723, 0, 7415, 0, -13331, 0, 41526, 65536, 41526, 0, -13331, 0, 7415, 0, -4723, 0, 3145, 0, -2112, 0, 1401, 0, -906, 0, 565, 0, -335, 0, 187, 0, -96, 0, 44, 0, -17, 0, 5]/(65536));
      | switch get_param(gcb, 'interp')
      |     case '1x'
      |         if ~strcmp(get_param([gcb, '/FIR 0'], 'Commented'), 'through')
      |             set_param([gcb, '/FIR 0'],'Commented','through');
      |         end
      |         
      |         if ~strcmp(get_param([gcb, '/FIR 1'], 'Commented'), 'through')
      |             set_param([gcb, '/FIR 1'],'Commented','through');
      |         end
      |         
      |         if ~strcmp(get_param([gcb, '/FIR 2'], 'Commented'), 'through')
      |             set_param([gcb, '/FIR 2'],'Commented','through');
      |         end
      |             
      |     case '2x'
      |         if ~strcmp(get_param([gcb, '/FIR 0'], 'Commented'), 'through')
      |             set_param([gcb, '/FIR 0'],'Commented','through');
      |         end
      |         
      |         if ~strcmp(get_param([gcb, '/FIR 1'], 'Commented'), 'through')
      |             set_param([gcb, '/FIR 1'],'Commented','through');
      |         end
      |         
      |         if ~strcmp(get_param([gcb, '/FIR 2'], 'Commented'), 'off')
      |             set_param([gcb, '/FIR 2'],'Commented','off');
      |         end
      | 
      |     case '4x'
      |         if ~strcmp(get_param([gcb, '/FIR 0'], 'Commented'), 'through')
      |             set_param([gcb, '/FIR 0'],'Commented','through');
      |         end
      |         
      |         if ~strcmp(get_param([gcb, '/FIR 1'], 'Commented'), 'off')
      |             set_param([gcb, '/FIR 1'],'Commented','off');
      |         end
      |         
      |         if ~strcmp(get_param([gcb, '/FIR 2'], 'Commented'), 'off')
      |             set_param([gcb, '/FIR 2'],'Commented','off');
      |         end
      |         
      |     case '8x'
      |         if ~strcmp(get_param([gcb, '/FIR 0'], 'Commented'), 'off')
      |             set_param([gcb, '/FIR 0'],'Commented','off');
      |         end
      |         
      |         if ~strcmp(get_param([gcb, '/FIR 1'], 'Commented'), 'off')
      |             set_param([gcb, '/FIR 1'],'Commented','off');
      |         end
      |         
      |         if ~strcmp(get_param([gcb, '/FIR 2'], 'Commented'), 'off')
      |             set_param([gcb, '/FIR 2'],'Commented','off');
      |         end
      | 
      | end
      mask TypeOptions interp: 1x | 2x | 4x | 8x
      mask DialogControl DescGroupVar Prompt: RF-DAC Interpolation Filter
      mask DialogControl DescTextVar Prompt: This block simulates the RF-DAC interpolation stage using the same coefficients stored in the interpolation filters.
      mask DialogControl ParameterGroupVar Prompt: Main
  NCO and Mixer : Subsystem
  Output Filter : Subsystem
  QMC Gain & Phase : Subsystem
  QMC Threshold : Subsystem
  RF-DAC : Subsystem
  Data Out : Outport  VectorParamsAs1DForOutWhenUnconnected=off
  wires:
  RF-DAC/1(Data Out) -> Data Out/1
  QMC Threshold/1(Data Out) -> RF-DAC/1(Data In)
  Output Filter/1(Data Out) -> QMC Threshold/1(Data In)
  Coarse Delay/1(Data Out) -> Output Filter/1(Data In)
  QMC Gain & Phase/1(Data Out) -> Coarse Delay/1(Data In)
  Data In/1 -> Interpolation Filter/1(Data In)
  NCO and Mixer/1(Data Out) -> QMC Gain & Phase/1(Data In)
  Interpolation Filter/1(Data Out) -> NCO and Mixer/1(Data In)

== system receiver/Time Synchronisation/Loop Filter ==
  note: Get centre of symbol
  note: The input to the loop filter should only be changed once per symbol.
      |
      | Use an enable register with the strobe from the NCC to hold the data in place.
  note: Get centre of symbol
  Real In : Inport
  Imag In : Inport  Port=2
  Signal In : Inport  Port=3
  Valid In : Inport  Port=4
  Reset : Inport  Port=5
  AddSub : xbsIndex_r4/AddSub  mode=Addition  use_carryin=off  use_carryout=off  en=off  latency=0  precision=User Defined  arith_type="Signed  (2's comp)"  n_bits=64  bin_pt=60  quantization=Truncate  overflow=Saturate  use_behavioral_HDL=off  hw_selection=Fabric  pipelined=off  dbl_ovrd=off  block_type=addsub
  AddSub1 : xbsIndex_r4/AddSub  mode=Addition  use_carryin=off  use_carryout=off  en=off  latency=0  precision=User Defined  arith_type="Signed  (2's comp)"  n_bits=64  bin_pt=60  quantization=Truncate  overflow=Saturate  use_behavioral_HDL=off  hw_selection=Fabric  pipelined=off  dbl_ovrd=off  block_type=addsub
  Delay1 : xbsIndex_r4/Delay  rst=off  infoeditControl=Selection of Reset will increase slice count due to use of real FFs and instead of SRLs  en=off  latency=32/2  reg_retiming=off  dbl_ovrd=off  block_type=delay
  Delay2 : xbsIndex_r4/Delay  rst=off  infoeditControl=Selection of Reset will increase slice count due to use of real FFs and instead of SRLs  en=off  latency=32/2  reg_retiming=off  dbl_ovrd=off  block_type=delay
  Delay3 : xbsIndex_r4/Delay  rst=off  infoeditControl=Selection of Reset will increase slice count due to use of real FFs and instead of SRLs  en=off  latency=32/2  reg_retiming=off  dbl_ovrd=off  block_type=delay
  K1_Gain : xbsIndex_r4/CMult  const=K1  gui_display_data_type=Fixed-point  const_n_bits=32  const_bin_pt=30  float_type=Single  exp_bits=8  fraction_bits=24  en=off  latency=0  precision=Full  arith_type="Signed  (2's comp)"  n_bits=3+28+16  bin_pt=28+16  quantization=Truncate  overflow=Wrap  use_behavioral_HDL=off  mem_type=Distributed RAM  pipeline=off  dbl_ovrd=off  block_type=cmult
  K2_Gain : xbsIndex_r4/CMult  const=K2  gui_display_data_type=Fixed-point  const_n_bits=32  const_bin_pt=30  float_type=Single  exp_bits=8  fraction_bits=24  en=off  latency=0  precision=Full  arith_type="Signed  (2's comp)"  n_bits=3+28+16  bin_pt=28+16  quantization=Truncate  overflow=Wrap  use_behavioral_HDL=off  mem_type=Distributed RAM  pipeline=off  dbl_ovrd=off  block_type=cmult
  Register : xbsIndex_r4/Register  init=0  rst=on  en=on  dbl_ovrd=off  block_type=register
  Register1 : xbsIndex_r4/Register  init=0  rst=on  en=on  dbl_ovrd=off  block_type=register
  Real Out : Outport  VectorParamsAs1DForOutWhenUnconnected=off
  Imag Out : Outport  Port=2  VectorParamsAs1DForOutWhenUnconnected=off
  Valid Out : Outport  Port=3  VectorParamsAs1DForOutWhenUnconnected=off
  Error Out : Outport  Port=4  VectorParamsAs1DForOutWhenUnconnected=off
  wires:
  Valid In/1 -> Register1/3, Delay3/1, Register/3
  AddSub1/1 -> Error Out/1
  Delay1/1 -> Real Out/1
  Delay2/1 -> Imag Out/1
  Register1/1 -> K2_Gain/1, K1_Gain/1
  Signal In/1 -> Register1/1
  Register/1 -> AddSub/2
  K1_Gain/1 -> AddSub1/1
  AddSub/1 -> AddSub1/2, Register/1
  Imag In/1 -> Delay2/1
  Real In/1 -> Delay1/1
  K2_Gain/1 -> AddSub/1
  Reset/1 -> Register1/2, Register/2
  Delay3/1 -> Valid Out/1

== system receiver/Time Synchronisation/NCC ==
  Error : Inport
  AddSub : xbsIndex_r4/AddSub  mode=Addition  use_carryin=off  use_carryout=off  en=off  latency=0  precision=User Defined  arith_type=Unsigned  n_bits=n+f  bin_pt=f  quantization=Truncate  overflow=Wrap  use_behavioral_HDL=off  hw_selection=Fabric  pipelined=off  dbl_ovrd=off  block_type=addsub
  AddSub1 : xbsIndex_r4/AddSub  mode=Addition  use_carryin=off  use_carryout=off  en=off  latency=0  precision=User Defined  arith_type="Signed  (2's comp)"  n_bits=n+f  bin_pt=f  quantization=Truncate  overflow=Saturate  use_behavioral_HDL=off  hw_selection=Fabric  pipelined=off  dbl_ovrd=off  block_type=addsub
  AddSub2 : xbsIndex_r4/AddSub  mode=Subtraction  use_carryin=off  use_carryout=off  en=off  latency=0  precision=User Defined  arith_type="Signed  (2's comp)"  n_bits=n+f  bin_pt=f  quantization=Truncate  overflow=Flag as error  use_behavioral_HDL=off  hw_selection=Fabric  pipelined=off  dbl_ovrd=off  block_type=addsub
  Constant : xbsIndex_r4/Constant  const=1  gui_display_data_type=Fixed-point  arith_type=Unsigned  n_bits=1  bin_pt=0  preci_type=Single  exp_width=8  frac_width=24  explicit_period=off  period=1  equ=P=C  opselect=C  inp2=PCIN>>17  opr=+  inp1=P  carry=CIN  dbl_ovrd=off  block_type=constant
  Constant1 : xbsIndex_r4/Constant  const=r  gui_display_data_type=Fixed-point  arith_type=Unsigned  n_bits=n  bin_pt=0  preci_type=Single  exp_width=8  frac_width=24  explicit_period=off  period=1  equ=P=C  opselect=C  inp2=PCIN>>17  opr=+  inp1=P  carry=CIN  dbl_ovrd=off  block_type=constant
  Mux : xbsIndex_r4/Mux  inputs=2  en=off  latency=0  precision=Full  arith_type=Unsigned  n_bits=16  bin_pt=14  quantization=Truncate  overflow=Wrap  dbl_ovrd=off  block_type=mux
  Register : xbsIndex_r4/Register  init=0  rst=off  en=off  dbl_ovrd=off  block_type=register
  Relational : xbsIndex_r4/Relational  mode=a>b  op_type=Bool  en=off  latency=0  dbl_ovrd=off  block_type=relational
  Relational1 : xbsIndex_r4/Relational  mode=a>b  op_type=Bool  en=off  latency=0  dbl_ovrd=off  block_type=relational
  Strobe : Outport  VectorParamsAs1DForOutWhenUnconnected=off
  wires:
  Constant/1 -> AddSub1/1
  Error/1 -> AddSub1/2
  Relational/1 -> Strobe/1
  AddSub1/1 -> AddSub/2
  Mux/1 -> AddSub/1
  Relational1/1 -> Mux/1
  AddSub2/1 -> Mux/3
  Constant1/1 -> Relational1/2, AddSub2/2
  Register/1 -> Relational/1, Relational1/1, Mux/2, AddSub2/1
  AddSub/1 -> Register/1, Relational/2

== system receiver/Time Synchronisation/Timing Error Detector ==
  Real In : Inport
  Imag In : Inport  Port=2
  AddSub : xbsIndex_r4/AddSub  mode=Subtraction  use_carryin=off  use_carryout=off  en=off  latency=0  precision=User Defined  arith_type="Signed  (2's comp)"  n_bits=31  bin_pt=30  quantization=Truncate  overflow=Saturate  use_behavioral_HDL=off  hw_selection=Fabric  pipelined=off  dbl_ovrd=off  block_type=addsub
  AddSub1 : xbsIndex_r4/AddSub  mode=Subtraction  use_carryin=off  use_carryout=off  en=off  latency=0  precision=User Defined  arith_type="Signed  (2's comp)"  n_bits=31  bin_pt=30  quantization=Truncate  overflow=Saturate  use_behavioral_HDL=off  hw_selection=Fabric  pipelined=off  dbl_ovrd=off  block_type=addsub
  AddSub2 : xbsIndex_r4/AddSub  mode=Addition  use_carryin=off  use_carryout=off  en=off  latency=0  precision=Full  arith_type="Signed  (2's comp)"  n_bits=16  bin_pt=13  quantization="Round  (unbiased: +/- Inf)"  overflow=Saturate  use_behavioral_HDL=off  hw_selection=Fabric  pipelined=off  dbl_ovrd=off  block_type=addsub
  Delay : xbsIndex_r4/Delay  rst=off  infoeditControl=Selection of Reset will increase slice count due to use of real FFs and instead of SRLs  en=off  latency=32  reg_retiming=off  dbl_ovrd=off  block_type=delay
  Delay1 : xbsIndex_r4/Delay  rst=off  infoeditControl=Selection of Reset will increase slice count due to use of real FFs and instead of SRLs  en=off  latency=32  reg_retiming=off  dbl_ovrd=off  block_type=delay
  Mult1 : xbsIndex_r4/Mult  precision=User Defined  arith_type=Unsigned  n_bits=31  bin_pt=30  quantization=Truncate  overflow=Saturate  en=off  latency=0  use_behavioral_HDL=off  opt=Speed  use_embedded=on  optimum_pipeline=off  pipeline=on  dbl_ovrd=off  use_rpm=on  placement_style=Triangular  block_type=mult
  Mult2 : xbsIndex_r4/Mult  precision=User Defined  arith_type=Unsigned  n_bits=31  bin_pt=30  quantization=Truncate  overflow=Saturate  en=off  latency=0  use_behavioral_HDL=off  opt=Speed  use_embedded=on  optimum_pipeline=off  pipeline=on  dbl_ovrd=off  use_rpm=on  placement_style=Triangular  block_type=mult
  Reinterpret : xbsIndex_r4/Reinterpret  force_arith_type=on  arith_type="Signed  (2's comp)"  force_bin_pt=on  bin_pt=15  block_type=reinterpret
  Reinterpret1 : xbsIndex_r4/Reinterpret  force_arith_type=on  arith_type="Signed  (2's comp)"  force_bin_pt=on  bin_pt=15  block_type=reinterpret
  Error : Outport  VectorParamsAs1DForOutWhenUnconnected=off
  wires:
  AddSub2/1 -> Error/1
  Reinterpret1/1 -> Mult1/2, Mult1/1
  Reinterpret/1 -> Mult2/1, Mult2/2
  Delay/1 -> AddSub/2
  Mult1/1 -> Delay/1, AddSub/1
  AddSub1/1 -> AddSub2/2
  Mult2/1 -> AddSub1/1, Delay1/1
  Delay1/1 -> AddSub1/2
  AddSub/1 -> AddSub2/1
  Imag In/1 -> Reinterpret/1
  Real In/1 -> Reinterpret1/1

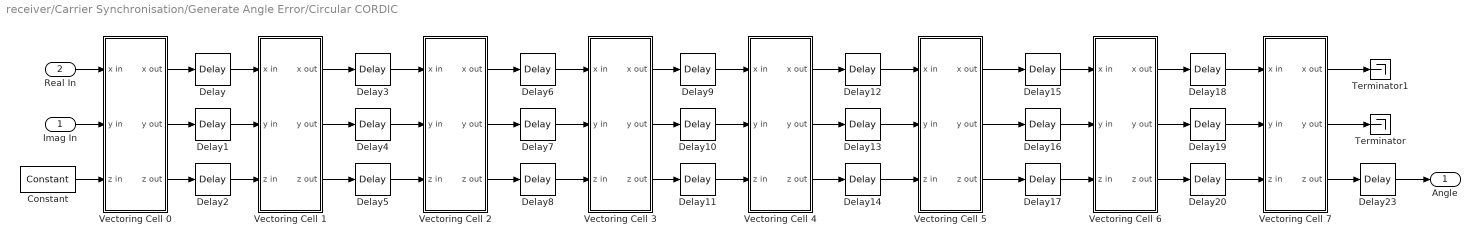
== system receiver/Carrier Synchronisation/Generate Angle Error/Circular CORDIC ==
  Imag In : Inport
  Real In : Inport  Port=2
  Constant : xbsIndex_r4/Constant  const=0  gui_display_data_type=Fixed-point  arith_type=Signed (2's comp)  n_bits=16  bin_pt=14  preci_type=Single  exp_width=8  frac_width=24  explicit_period=off  period=1  equ=P=C  opselect=C  inp2=PCIN>>17  opr=+  inp1=P  carry=CIN  dbl_ovrd=off  block_type=constant
  Delay{,1..20,23} (22 alike) : xbsIndex_r4/Delay  rst=off  infoeditControl=Selection of Reset will increase slice count due to use of real FFs and instead of SRLs  en=off  latency=1  reg_retiming=off  dbl_ovrd=off  block_type=delay
  Terminator : Terminator
  Terminator1 : Terminator
  Vectoring Cell 0 : Subsystem  mask(Cordic Vectoring Cell){i=0}
      mask prompts: i "Iteration:"
      mask help: some notes to go here
      mask DialogControl DescGroupVar Prompt: CORDIC Vectoring Cell
      mask DialogControl DescTextVar Prompt: A single cell of a vectoring CORDIC unrolled architecture.
      mask DialogControl ParameterGroupVar Prompt: Main
  Vectoring Cell 1 : Subsystem  mask(Cordic Vectoring Cell){i=1}
      mask prompts: i "Iteration:"
      mask help: some notes to go here
      mask DialogControl DescGroupVar Prompt: CORDIC Vectoring Cell
      mask DialogControl DescTextVar Prompt: A single cell of a vectoring CORDIC unrolled architecture.
      mask DialogControl ParameterGroupVar Prompt: Main
  Vectoring Cell 2 : Subsystem  mask(Cordic Vectoring Cell){i=2}
      mask prompts: i "Iteration:"
      mask help: some notes to go here
      mask DialogControl DescGroupVar Prompt: CORDIC Vectoring Cell
      mask DialogControl DescTextVar Prompt: A single cell of a vectoring CORDIC unrolled architecture.
      mask DialogControl ParameterGroupVar Prompt: Main
  Vectoring Cell 3 : Subsystem  mask(Cordic Vectoring Cell){i=3}
      mask prompts: i "Iteration:"
      mask help: some notes to go here
      mask DialogControl DescGroupVar Prompt: CORDIC Vectoring Cell
      mask DialogControl DescTextVar Prompt: A single cell of a vectoring CORDIC unrolled architecture.
      mask DialogControl ParameterGroupVar Prompt: Main
  Vectoring Cell 4 : Subsystem  mask(Cordic Vectoring Cell){i=4}
      mask prompts: i "Iteration:"
      mask help: some notes to go here
      mask DialogControl DescGroupVar Prompt: CORDIC Vectoring Cell
      mask DialogControl DescTextVar Prompt: A single cell of a vectoring CORDIC unrolled architecture.
      mask DialogControl ParameterGroupVar Prompt: Main
  Vectoring Cell 5 : Subsystem  mask(Cordic Vectoring Cell){i=5}
      mask prompts: i "Iteration:"
      mask help: some notes to go here
      mask DialogControl DescGroupVar Prompt: CORDIC Vectoring Cell
      mask DialogControl DescTextVar Prompt: A single cell of a vectoring CORDIC unrolled architecture.
      mask DialogControl ParameterGroupVar Prompt: Main
  Vectoring Cell 6 : Subsystem  mask(Cordic Vectoring Cell){i=6}
      mask prompts: i "Iteration:"
      mask help: some notes to go here
      mask DialogControl DescGroupVar Prompt: CORDIC Vectoring Cell
      mask DialogControl DescTextVar Prompt: A single cell of a vectoring CORDIC unrolled architecture.
      mask DialogControl ParameterGroupVar Prompt: Main
  Vectoring Cell 7 : Subsystem  mask(Cordic Vectoring Cell){i=7}
      mask prompts: i "Iteration:"
      mask help: some notes to go here
      mask DialogControl DescGroupVar Prompt: CORDIC Vectoring Cell
      mask DialogControl DescTextVar Prompt: A single cell of a vectoring CORDIC unrolled architecture.
      mask DialogControl ParameterGroupVar Prompt: Main
  Angle : Outport  VectorParamsAs1DForOutWhenUnconnected=off
  wires:
  Vectoring Cell 7/1(x out) -> Terminator1/1
  Vectoring Cell 7/2(y out) -> Terminator/1
  Delay23/1 -> Angle/1
  Constant/1 -> Vectoring Cell 0/3(z in)
  Imag In/1 -> Vectoring Cell 0/2(y in)
  Real In/1 -> Vectoring Cell 0/1(x in)
  Vectoring Cell 7/3(z out) -> Delay23/1
  Delay11/1 -> Vectoring Cell 4/3(z in)
  Delay17/1 -> Vectoring Cell 6/3(z in)
  Vectoring Cell 5/3(z out) -> Delay17/1
  Delay2/1 -> Vectoring Cell 1/3(z in)
  Vectoring Cell 4/1(x out) -> Delay12/1
  Vectoring Cell 4/2(y out) -> Delay13/1
  Delay12/1 -> Vectoring Cell 5/1(x in)
  Vectoring Cell 0/2(y out) -> Delay1/1
  Vectoring Cell 6/1(x out) -> Delay18/1
  Vectoring Cell 2/3(z out) -> Delay8/1
  Vectoring Cell 0/1(x out) -> Delay/1
  Vectoring Cell 5/2(y out) -> Delay16/1
  Delay/1 -> Vectoring Cell 1/1(x in)
  Vectoring Cell 5/1(x out) -> Delay15/1
  Vectoring Cell 1/2(y out) -> Delay4/1
  Vectoring Cell 3/2(y out) -> Delay10/1
  Delay8/1 -> Vectoring Cell 3/3(z in)
  Vectoring Cell 4/3(z out) -> Delay14/1
  Delay3/1 -> Vectoring Cell 2/1(x in)
  Delay4/1 -> Vectoring Cell 2/2(y in)
  Delay19/1 -> Vectoring Cell 7/2(y in)
  Delay6/1 -> Vectoring Cell 3/1(x in)
  Vectoring Cell 3/3(z out) -> Delay11/1
  Vectoring Cell 2/2(y out) -> Delay7/1
  Delay10/1 -> Vectoring Cell 4/2(y in)
  Vectoring Cell 0/3(z out) -> Delay2/1
  Delay18/1 -> Vectoring Cell 7/1(x in)
  Delay16/1 -> Vectoring Cell 6/2(y in)
  Vectoring Cell 1/1(x out) -> Delay3/1
  Delay9/1 -> Vectoring Cell 4/1(x in)
  Delay13/1 -> Vectoring Cell 5/2(y in)
  Vectoring Cell 3/1(x out) -> Delay9/1
  Delay1/1 -> Vectoring Cell 1/2(y in)
  Delay7/1 -> Vectoring Cell 3/2(y in)
  Delay15/1 -> Vectoring Cell 6/1(x in)
  Delay20/1 -> Vectoring Cell 7/3(z in)
  Delay14/1 -> Vectoring Cell 5/3(z in)
  Vectoring Cell 1/3(z out) -> Delay5/1
  Vectoring Cell 2/1(x out) -> Delay6/1
  Vectoring Cell 6/2(y out) -> Delay19/1
  Delay5/1 -> Vectoring Cell 2/3(z in)
  Vectoring Cell 6/3(z out) -> Delay20/1
